simulink library "csc_stm_simplified_temperature_model_collection_lib"  (R2014b)
settings: Solver=ode45  StartTime=0.0  StopTime=10.0  RelTol=1e-3
undefined symbols (not defined in the file or in its folder): stm_celcius_to_bits_slope, stm_tc10_eqn_coefficients, stm_tc11_eqn_coefficients, stm_tc12_eqn_coefficients, stm_tc13_eqn_coefficients, stm_tc14_eqn_coefficients, stm_tc15_eqn_coefficients, stm_tc16_eqn_coefficients, stm_tc17_eqn_coefficients, stm_tc18_eqn_coefficients, stm_tc19_eqn_coefficients, stm_tc1_eqn_coefficients, stm_tc20_eqn_coefficients, stm_tc21_eqn_coefficients, stm_tc22_eqn_coefficients, stm_tc23_eqn_coefficients, stm_tc24_eqn_coefficients, stm_tc25_eqn_coefficients, stm_tc26_eqn_coefficients, stm_tc27_eqn_coefficients, stm_tc28_eqn_coefficients, stm_tc29_eqn_coefficients, stm_tc2_eqn_coefficients, stm_tc30_eqn_coefficients, stm_tc31_eqn_coefficients, stm_tc32_eqn_coefficients, stm_tc33_eqn_coefficients, stm_tc34_eqn_coefficients, stm_tc35_eqn_coefficients, stm_tc36_eqn_coefficients, stm_tc37_eqn_coefficients, stm_tc38_eqn_coefficients, stm_tc39_eqn_coefficients, stm_tc3_eqn_coefficients, stm_tc40_eqn_coefficients, stm_tc41_eqn_coefficients, stm_tc42_eqn_coefficients, stm_tc43_eqn_coefficients, stm_tc44_eqn_coefficients, stm_tc45_eqn_coefficients, stm_tc46_eqn_coefficients, stm_tc47_eqn_coefficients, stm_tc48_eqn_coefficients, stm_tc49_eqn_coefficients, stm_tc4_eqn_coefficients, stm_tc50_eqn_coefficients, stm_tc51_eqn_coefficients, stm_tc52_eqn_coefficients, stm_tc53_eqn_coefficients, stm_tc54_eqn_coefficients, stm_tc55_eqn_coefficients, stm_tc56_eqn_coefficients, stm_tc57_eqn_coefficients, stm_tc58_eqn_coefficients, stm_tc59_eqn_coefficients, stm_tc5_eqn_coefficients, stm_tc60_eqn_coefficients, stm_tc61_eqn_coefficients, stm_tc62_eqn_coefficients, stm_tc63_eqn_coefficients ... (+5)
libraries: csu_stm_simplified_temperature_model_lib x64, util_info_lib x1
settings Model: Creator=escrane  LastModifiedBy=mstewart

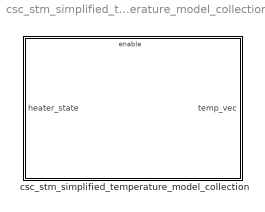
== system csc_stm_simplified_temperature_model_collection_lib ==
  csc_stm_simplified_temperature_model_collection : Subsystem
      mask Display: color('blue');text(0.05, 0.02, 'MoonEx', 'HorizontalAlignment', 'Left', 'VerticalAlignment', 'Bottom');color('red');text(0.95, 0.02, 'Autogenerated', 'HorizontalAlignment', 'Right', 'VerticalAlignment', 'Bottom');

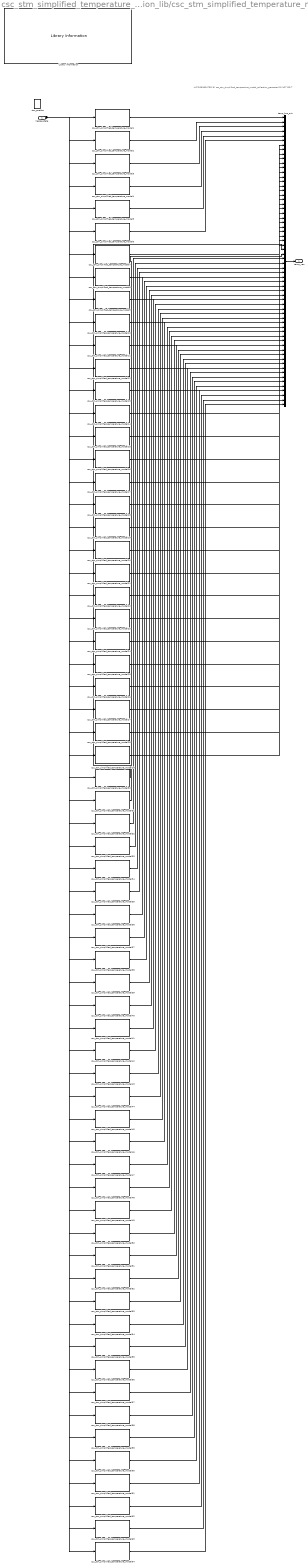
== system csc_stm_simplified_temperature_model_collection_lib/csc_stm_simplified_temperature_model_collection ==
  note: AUTOGENERATED BY csc_stm_simplified_temperature_model_collection_generate
      | DO NOT EDIT
  heater_state : Inport
  stm_enable : EnablePort
  Library Information : util_info_lib/Library Information  owner='NONE'
  csu_stm_simplified_temperature_model1 : csu_stm_simplified_temperature_model_lib/csu_stm_simplified_temperature_model  tc_idx=1  heater_idx=stm_tc1_heater_id  initial_temperature=stm_tc1_initial_temperature  min_temperature=-25  max_temperature=+105  C1=stm_tc1_eqn_coefficients(1)  C2=stm_tc1_eqn_coefficients(2)  C3=stm_tc1_eqn_coefficients(3)  C4=stm_tc1_eqn_coefficients(4)  heater_power=stm_tc1_eqn_coefficients(5)  slope=stm_celcius_to_bits_slope  offset=stm_celcius_to_bits_offset
  csu_stm_simplified_temperature_model10 : csu_stm_simplified_temperature_model_lib/csu_stm_simplified_temperature_model  tc_idx=10  heater_idx=stm_tc10_heater_id  initial_temperature=stm_tc10_initial_temperature  min_temperature=-25  max_temperature=+105  C1=stm_tc10_eqn_coefficients(1)  C2=stm_tc10_eqn_coefficients(2)  C3=stm_tc10_eqn_coefficients(3)  C4=stm_tc10_eqn_coefficients(4)  heater_power=stm_tc10_eqn_coefficients(5)  slope=stm_celcius_to_bits_slope  offset=stm_celcius_to_bits_offset
  csu_stm_simplified_temperature_model11 : csu_stm_simplified_temperature_model_lib/csu_stm_simplified_temperature_model  tc_idx=11  heater_idx=stm_tc11_heater_id  initial_temperature=stm_tc11_initial_temperature  min_temperature=-25  max_temperature=+105  C1=stm_tc11_eqn_coefficients(1)  C2=stm_tc11_eqn_coefficients(2)  C3=stm_tc11_eqn_coefficients(3)  C4=stm_tc11_eqn_coefficients(4)  heater_power=stm_tc11_eqn_coefficients(5)  slope=stm_celcius_to_bits_slope  offset=stm_celcius_to_bits_offset
  csu_stm_simplified_temperature_model12 : csu_stm_simplified_temperature_model_lib/csu_stm_simplified_temperature_model  tc_idx=12  heater_idx=stm_tc12_heater_id  initial_temperature=stm_tc12_initial_temperature  min_temperature=-25  max_temperature=+105  C1=stm_tc12_eqn_coefficients(1)  C2=stm_tc12_eqn_coefficients(2)  C3=stm_tc12_eqn_coefficients(3)  C4=stm_tc12_eqn_coefficients(4)  heater_power=stm_tc12_eqn_coefficients(5)  slope=stm_celcius_to_bits_slope  offset=stm_celcius_to_bits_offset
  csu_stm_simplified_temperature_model13 : csu_stm_simplified_temperature_model_lib/csu_stm_simplified_temperature_model  tc_idx=13  heater_idx=stm_tc13_heater_id  initial_temperature=stm_tc13_initial_temperature  min_temperature=-25  max_temperature=+105  C1=stm_tc13_eqn_coefficients(1)  C2=stm_tc13_eqn_coefficients(2)  C3=stm_tc13_eqn_coefficients(3)  C4=stm_tc13_eqn_coefficients(4)  heater_power=stm_tc13_eqn_coefficients(5)  slope=stm_celcius_to_bits_slope  offset=stm_celcius_to_bits_offset
  csu_stm_simplified_temperature_model14 : csu_stm_simplified_temperature_model_lib/csu_stm_simplified_temperature_model  tc_idx=14  heater_idx=stm_tc14_heater_id  initial_temperature=stm_tc14_initial_temperature  min_temperature=-25  max_temperature=+105  C1=stm_tc14_eqn_coefficients(1)  C2=stm_tc14_eqn_coefficients(2)  C3=stm_tc14_eqn_coefficients(3)  C4=stm_tc14_eqn_coefficients(4)  heater_power=stm_tc14_eqn_coefficients(5)  slope=stm_celcius_to_bits_slope  offset=stm_celcius_to_bits_offset
  csu_stm_simplified_temperature_model15 : csu_stm_simplified_temperature_model_lib/csu_stm_simplified_temperature_model  tc_idx=15  heater_idx=stm_tc15_heater_id  initial_temperature=stm_tc15_initial_temperature  min_temperature=-25  max_temperature=+105  C1=stm_tc15_eqn_coefficients(1)  C2=stm_tc15_eqn_coefficients(2)  C3=stm_tc15_eqn_coefficients(3)  C4=stm_tc15_eqn_coefficients(4)  heater_power=stm_tc15_eqn_coefficients(5)  slope=stm_celcius_to_bits_slope  offset=stm_celcius_to_bits_offset
  csu_stm_simplified_temperature_model16 : csu_stm_simplified_temperature_model_lib/csu_stm_simplified_temperature_model  tc_idx=16  heater_idx=stm_tc16_heater_id  initial_temperature=stm_tc16_initial_temperature  min_temperature=-25  max_temperature=+105  C1=stm_tc16_eqn_coefficients(1)  C2=stm_tc16_eqn_coefficients(2)  C3=stm_tc16_eqn_coefficients(3)  C4=stm_tc16_eqn_coefficients(4)  heater_power=stm_tc16_eqn_coefficients(5)  slope=stm_celcius_to_bits_slope  offset=stm_celcius_to_bits_offset
  csu_stm_simplified_temperature_model17 : csu_stm_simplified_temperature_model_lib/csu_stm_simplified_temperature_model  tc_idx=17  heater_idx=stm_tc17_heater_id  initial_temperature=stm_tc17_initial_temperature  min_temperature=-25  max_temperature=+105  C1=stm_tc17_eqn_coefficients(1)  C2=stm_tc17_eqn_coefficients(2)  C3=stm_tc17_eqn_coefficients(3)  C4=stm_tc17_eqn_coefficients(4)  heater_power=stm_tc17_eqn_coefficients(5)  slope=stm_celcius_to_bits_slope  offset=stm_celcius_to_bits_offset
  csu_stm_simplified_temperature_model18 : csu_stm_simplified_temperature_model_lib/csu_stm_simplified_temperature_model  tc_idx=18  heater_idx=stm_tc18_heater_id  initial_temperature=stm_tc18_initial_temperature  min_temperature=-25  max_temperature=+105  C1=stm_tc18_eqn_coefficients(1)  C2=stm_tc18_eqn_coefficients(2)  C3=stm_tc18_eqn_coefficients(3)  C4=stm_tc18_eqn_coefficients(4)  heater_power=stm_tc18_eqn_coefficients(5)  slope=stm_celcius_to_bits_slope  offset=stm_celcius_to_bits_offset
  csu_stm_simplified_temperature_model19 : csu_stm_simplified_temperature_model_lib/csu_stm_simplified_temperature_model  tc_idx=19  heater_idx=stm_tc19_heater_id  initial_temperature=stm_tc19_initial_temperature  min_temperature=-25  max_temperature=+105  C1=stm_tc19_eqn_coefficients(1)  C2=stm_tc19_eqn_coefficients(2)  C3=stm_tc19_eqn_coefficients(3)  C4=stm_tc19_eqn_coefficients(4)  heater_power=stm_tc19_eqn_coefficients(5)  slope=stm_celcius_to_bits_slope  offset=stm_celcius_to_bits_offset
  csu_stm_simplified_temperature_model2 : csu_stm_simplified_temperature_model_lib/csu_stm_simplified_temperature_model  tc_idx=2  heater_idx=stm_tc2_heater_id  initial_temperature=stm_tc2_initial_temperature  min_temperature=-25  max_temperature=+105  C1=stm_tc2_eqn_coefficients(1)  C2=stm_tc2_eqn_coefficients(2)  C3=stm_tc2_eqn_coefficients(3)  C4=stm_tc2_eqn_coefficients(4)  heater_power=stm_tc2_eqn_coefficients(5)  slope=stm_celcius_to_bits_slope  offset=stm_celcius_to_bits_offset
  csu_stm_simplified_temperature_model20 : csu_stm_simplified_temperature_model_lib/csu_stm_simplified_temperature_model  tc_idx=20  heater_idx=stm_tc20_heater_id  initial_temperature=stm_tc20_initial_temperature  min_temperature=-25  max_temperature=+105  C1=stm_tc20_eqn_coefficients(1)  C2=stm_tc20_eqn_coefficients(2)  C3=stm_tc20_eqn_coefficients(3)  C4=stm_tc20_eqn_coefficients(4)  heater_power=stm_tc20_eqn_coefficients(5)  slope=stm_celcius_to_bits_slope  offset=stm_celcius_to_bits_offset
  csu_stm_simplified_temperature_model21 : csu_stm_simplified_temperature_model_lib/csu_stm_simplified_temperature_model  tc_idx=21  heater_idx=stm_tc21_heater_id  initial_temperature=stm_tc21_initial_temperature  min_temperature=-25  max_temperature=+105  C1=stm_tc21_eqn_coefficients(1)  C2=stm_tc21_eqn_coefficients(2)  C3=stm_tc21_eqn_coefficients(3)  C4=stm_tc21_eqn_coefficients(4)  heater_power=stm_tc21_eqn_coefficients(5)  slope=stm_celcius_to_bits_slope  offset=stm_celcius_to_bits_offset
  csu_stm_simplified_temperature_model22 : csu_stm_simplified_temperature_model_lib/csu_stm_simplified_temperature_model  tc_idx=22  heater_idx=stm_tc22_heater_id  initial_temperature=stm_tc22_initial_temperature  min_temperature=-25  max_temperature=+105  C1=stm_tc22_eqn_coefficients(1)  C2=stm_tc22_eqn_coefficients(2)  C3=stm_tc22_eqn_coefficients(3)  C4=stm_tc22_eqn_coefficients(4)  heater_power=stm_tc22_eqn_coefficients(5)  slope=stm_celcius_to_bits_slope  offset=stm_celcius_to_bits_offset
  csu_stm_simplified_temperature_model23 : csu_stm_simplified_temperature_model_lib/csu_stm_simplified_temperature_model  tc_idx=23  heater_idx=stm_tc23_heater_id  initial_temperature=stm_tc23_initial_temperature  min_temperature=-25  max_temperature=+105  C1=stm_tc23_eqn_coefficients(1)  C2=stm_tc23_eqn_coefficients(2)  C3=stm_tc23_eqn_coefficients(3)  C4=stm_tc23_eqn_coefficients(4)  heater_power=stm_tc23_eqn_coefficients(5)  slope=stm_celcius_to_bits_slope  offset=stm_celcius_to_bits_offset
  csu_stm_simplified_temperature_model24 : csu_stm_simplified_temperature_model_lib/csu_stm_simplified_temperature_model  tc_idx=24  heater_idx=stm_tc24_heater_id  initial_temperature=stm_tc24_initial_temperature  min_temperature=-25  max_temperature=+105  C1=stm_tc24_eqn_coefficients(1)  C2=stm_tc24_eqn_coefficients(2)  C3=stm_tc24_eqn_coefficients(3)  C4=stm_tc24_eqn_coefficients(4)  heater_power=stm_tc24_eqn_coefficients(5)  slope=stm_celcius_to_bits_slope  offset=stm_celcius_to_bits_offset
  csu_stm_simplified_temperature_model25 : csu_stm_simplified_temperature_model_lib/csu_stm_simplified_temperature_model  tc_idx=25  heater_idx=stm_tc25_heater_id  initial_temperature=stm_tc25_initial_temperature  min_temperature=-25  max_temperature=+105  C1=stm_tc25_eqn_coefficients(1)  C2=stm_tc25_eqn_coefficients(2)  C3=stm_tc25_eqn_coefficients(3)  C4=stm_tc25_eqn_coefficients(4)  heater_power=stm_tc25_eqn_coefficients(5)  slope=stm_celcius_to_bits_slope  offset=stm_celcius_to_bits_offset
  csu_stm_simplified_temperature_model26 : csu_stm_simplified_temperature_model_lib/csu_stm_simplified_temperature_model  tc_idx=26  heater_idx=stm_tc26_heater_id  initial_temperature=stm_tc26_initial_temperature  min_temperature=-25  max_temperature=+105  C1=stm_tc26_eqn_coefficients(1)  C2=stm_tc26_eqn_coefficients(2)  C3=stm_tc26_eqn_coefficients(3)  C4=stm_tc26_eqn_coefficients(4)  heater_power=stm_tc26_eqn_coefficients(5)  slope=stm_celcius_to_bits_slope  offset=stm_celcius_to_bits_offset
  csu_stm_simplified_temperature_model27 : csu_stm_simplified_temperature_model_lib/csu_stm_simplified_temperature_model  tc_idx=27  heater_idx=stm_tc27_heater_id  initial_temperature=stm_tc27_initial_temperature  min_temperature=-25  max_temperature=+105  C1=stm_tc27_eqn_coefficients(1)  C2=stm_tc27_eqn_coefficients(2)  C3=stm_tc27_eqn_coefficients(3)  C4=stm_tc27_eqn_coefficients(4)  heater_power=stm_tc27_eqn_coefficients(5)  slope=stm_celcius_to_bits_slope  offset=stm_celcius_to_bits_offset
  csu_stm_simplified_temperature_model28 : csu_stm_simplified_temperature_model_lib/csu_stm_simplified_temperature_model  tc_idx=28  heater_idx=stm_tc28_heater_id  initial_temperature=stm_tc28_initial_temperature  min_temperature=-25  max_temperature=+105  C1=stm_tc28_eqn_coefficients(1)  C2=stm_tc28_eqn_coefficients(2)  C3=stm_tc28_eqn_coefficients(3)  C4=stm_tc28_eqn_coefficients(4)  heater_power=stm_tc28_eqn_coefficients(5)  slope=stm_celcius_to_bits_slope  offset=stm_celcius_to_bits_offset
  csu_stm_simplified_temperature_model29 : csu_stm_simplified_temperature_model_lib/csu_stm_simplified_temperature_model  tc_idx=29  heater_idx=stm_tc29_heater_id  initial_temperature=stm_tc29_initial_temperature  min_temperature=-25  max_temperature=+105  C1=stm_tc29_eqn_coefficients(1)  C2=stm_tc29_eqn_coefficients(2)  C3=stm_tc29_eqn_coefficients(3)  C4=stm_tc29_eqn_coefficients(4)  heater_power=stm_tc29_eqn_coefficients(5)  slope=stm_celcius_to_bits_slope  offset=stm_celcius_to_bits_offset
  csu_stm_simplified_temperature_model3 : csu_stm_simplified_temperature_model_lib/csu_stm_simplified_temperature_model  tc_idx=3  heater_idx=stm_tc3_heater_id  initial_temperature=stm_tc3_initial_temperature  min_temperature=-25  max_temperature=+105  C1=stm_tc3_eqn_coefficients(1)  C2=stm_tc3_eqn_coefficients(2)  C3=stm_tc3_eqn_coefficients(3)  C4=stm_tc3_eqn_coefficients(4)  heater_power=stm_tc3_eqn_coefficients(5)  slope=stm_celcius_to_bits_slope  offset=stm_celcius_to_bits_offset
  csu_stm_simplified_temperature_model30 : csu_stm_simplified_temperature_model_lib/csu_stm_simplified_temperature_model  tc_idx=30  heater_idx=stm_tc30_heater_id  initial_temperature=stm_tc30_initial_temperature  min_temperature=-25  max_temperature=+105  C1=stm_tc30_eqn_coefficients(1)  C2=stm_tc30_eqn_coefficients(2)  C3=stm_tc30_eqn_coefficients(3)  C4=stm_tc30_eqn_coefficients(4)  heater_power=stm_tc30_eqn_coefficients(5)  slope=stm_celcius_to_bits_slope  offset=stm_celcius_to_bits_offset
  csu_stm_simplified_temperature_model31 : csu_stm_simplified_temperature_model_lib/csu_stm_simplified_temperature_model  tc_idx=31  heater_idx=stm_tc31_heater_id  initial_temperature=stm_tc31_initial_temperature  min_temperature=-25  max_temperature=+105  C1=stm_tc31_eqn_coefficients(1)  C2=stm_tc31_eqn_coefficients(2)  C3=stm_tc31_eqn_coefficients(3)  C4=stm_tc31_eqn_coefficients(4)  heater_power=stm_tc31_eqn_coefficients(5)  slope=stm_celcius_to_bits_slope  offset=stm_celcius_to_bits_offset
  csu_stm_simplified_temperature_model32 : csu_stm_simplified_temperature_model_lib/csu_stm_simplified_temperature_model  tc_idx=32  heater_idx=stm_tc32_heater_id  initial_temperature=stm_tc32_initial_temperature  min_temperature=-25  max_temperature=+105  C1=stm_tc32_eqn_coefficients(1)  C2=stm_tc32_eqn_coefficients(2)  C3=stm_tc32_eqn_coefficients(3)  C4=stm_tc32_eqn_coefficients(4)  heater_power=stm_tc32_eqn_coefficients(5)  slope=stm_celcius_to_bits_slope  offset=stm_celcius_to_bits_offset
  csu_stm_simplified_temperature_model33 : csu_stm_simplified_temperature_model_lib/csu_stm_simplified_temperature_model  tc_idx=33  heater_idx=stm_tc33_heater_id  initial_temperature=stm_tc33_initial_temperature  min_temperature=-25  max_temperature=+105  C1=stm_tc33_eqn_coefficients(1)  C2=stm_tc33_eqn_coefficients(2)  C3=stm_tc33_eqn_coefficients(3)  C4=stm_tc33_eqn_coefficients(4)  heater_power=stm_tc33_eqn_coefficients(5)  slope=stm_celcius_to_bits_slope  offset=stm_celcius_to_bits_offset
  csu_stm_simplified_temperature_model34 : csu_stm_simplified_temperature_model_lib/csu_stm_simplified_temperature_model  tc_idx=34  heater_idx=stm_tc34_heater_id  initial_temperature=stm_tc34_initial_temperature  min_temperature=-25  max_temperature=+105  C1=stm_tc34_eqn_coefficients(1)  C2=stm_tc34_eqn_coefficients(2)  C3=stm_tc34_eqn_coefficients(3)  C4=stm_tc34_eqn_coefficients(4)  heater_power=stm_tc34_eqn_coefficients(5)  slope=stm_celcius_to_bits_slope  offset=stm_celcius_to_bits_offset
  csu_stm_simplified_temperature_model35 : csu_stm_simplified_temperature_model_lib/csu_stm_simplified_temperature_model  tc_idx=35  heater_idx=stm_tc35_heater_id  initial_temperature=stm_tc35_initial_temperature  min_temperature=-25  max_temperature=+105  C1=stm_tc35_eqn_coefficients(1)  C2=stm_tc35_eqn_coefficients(2)  C3=stm_tc35_eqn_coefficients(3)  C4=stm_tc35_eqn_coefficients(4)  heater_power=stm_tc35_eqn_coefficients(5)  slope=stm_celcius_to_bits_slope  offset=stm_celcius_to_bits_offset
  csu_stm_simplified_temperature_model36 : csu_stm_simplified_temperature_model_lib/csu_stm_simplified_temperature_model  tc_idx=36  heater_idx=stm_tc36_heater_id  initial_temperature=stm_tc36_initial_temperature  min_temperature=-25  max_temperature=+105  C1=stm_tc36_eqn_coefficients(1)  C2=stm_tc36_eqn_coefficients(2)  C3=stm_tc36_eqn_coefficients(3)  C4=stm_tc36_eqn_coefficients(4)  heater_power=stm_tc36_eqn_coefficients(5)  slope=stm_celcius_to_bits_slope  offset=stm_celcius_to_bits_offset
  csu_stm_simplified_temperature_model37 : csu_stm_simplified_temperature_model_lib/csu_stm_simplified_temperature_model  tc_idx=37  heater_idx=stm_tc37_heater_id  initial_temperature=stm_tc37_initial_temperature  min_temperature=-25  max_temperature=+105  C1=stm_tc37_eqn_coefficients(1)  C2=stm_tc37_eqn_coefficients(2)  C3=stm_tc37_eqn_coefficients(3)  C4=stm_tc37_eqn_coefficients(4)  heater_power=stm_tc37_eqn_coefficients(5)  slope=stm_celcius_to_bits_slope  offset=stm_celcius_to_bits_offset
  csu_stm_simplified_temperature_model38 : csu_stm_simplified_temperature_model_lib/csu_stm_simplified_temperature_model  tc_idx=38  heater_idx=stm_tc38_heater_id  initial_temperature=stm_tc38_initial_temperature  min_temperature=-25  max_temperature=+105  C1=stm_tc38_eqn_coefficients(1)  C2=stm_tc38_eqn_coefficients(2)  C3=stm_tc38_eqn_coefficients(3)  C4=stm_tc38_eqn_coefficients(4)  heater_power=stm_tc38_eqn_coefficients(5)  slope=stm_celcius_to_bits_slope  offset=stm_celcius_to_bits_offset
  csu_stm_simplified_temperature_model39 : csu_stm_simplified_temperature_model_lib/csu_stm_simplified_temperature_model  tc_idx=39  heater_idx=stm_tc39_heater_id  initial_temperature=stm_tc39_initial_temperature  min_temperature=-25  max_temperature=+105  C1=stm_tc39_eqn_coefficients(1)  C2=stm_tc39_eqn_coefficients(2)  C3=stm_tc39_eqn_coefficients(3)  C4=stm_tc39_eqn_coefficients(4)  heater_power=stm_tc39_eqn_coefficients(5)  slope=stm_celcius_to_bits_slope  offset=stm_celcius_to_bits_offset
  csu_stm_simplified_temperature_model4 : csu_stm_simplified_temperature_model_lib/csu_stm_simplified_temperature_model  tc_idx=4  heater_idx=stm_tc4_heater_id  initial_temperature=stm_tc4_initial_temperature  min_temperature=-25  max_temperature=+105  C1=stm_tc4_eqn_coefficients(1)  C2=stm_tc4_eqn_coefficients(2)  C3=stm_tc4_eqn_coefficients(3)  C4=stm_tc4_eqn_coefficients(4)  heater_power=stm_tc4_eqn_coefficients(5)  slope=stm_celcius_to_bits_slope  offset=stm_celcius_to_bits_offset
  csu_stm_simplified_temperature_model40 : csu_stm_simplified_temperature_model_lib/csu_stm_simplified_temperature_model  tc_idx=40  heater_idx=stm_tc40_heater_id  initial_temperature=stm_tc40_initial_temperature  min_temperature=-25  max_temperature=+105  C1=stm_tc40_eqn_coefficients(1)  C2=stm_tc40_eqn_coefficients(2)  C3=stm_tc40_eqn_coefficients(3)  C4=stm_tc40_eqn_coefficients(4)  heater_power=stm_tc40_eqn_coefficients(5)  slope=stm_celcius_to_bits_slope  offset=stm_celcius_to_bits_offset
  csu_stm_simplified_temperature_model41 : csu_stm_simplified_temperature_model_lib/csu_stm_simplified_temperature_model  tc_idx=41  heater_idx=stm_tc41_heater_id  initial_temperature=stm_tc41_initial_temperature  min_temperature=-25  max_temperature=+105  C1=stm_tc41_eqn_coefficients(1)  C2=stm_tc41_eqn_coefficients(2)  C3=stm_tc41_eqn_coefficients(3)  C4=stm_tc41_eqn_coefficients(4)  heater_power=stm_tc41_eqn_coefficients(5)  slope=stm_celcius_to_bits_slope  offset=stm_celcius_to_bits_offset
  csu_stm_simplified_temperature_model42 : csu_stm_simplified_temperature_model_lib/csu_stm_simplified_temperature_model  tc_idx=42  heater_idx=stm_tc42_heater_id  initial_temperature=stm_tc42_initial_temperature  min_temperature=-25  max_temperature=+105  C1=stm_tc42_eqn_coefficients(1)  C2=stm_tc42_eqn_coefficients(2)  C3=stm_tc42_eqn_coefficients(3)  C4=stm_tc42_eqn_coefficients(4)  heater_power=stm_tc42_eqn_coefficients(5)  slope=stm_celcius_to_bits_slope  offset=stm_celcius_to_bits_offset
  csu_stm_simplified_temperature_model43 : csu_stm_simplified_temperature_model_lib/csu_stm_simplified_temperature_model  tc_idx=43  heater_idx=stm_tc43_heater_id  initial_temperature=stm_tc43_initial_temperature  min_temperature=-25  max_temperature=+105  C1=stm_tc43_eqn_coefficients(1)  C2=stm_tc43_eqn_coefficients(2)  C3=stm_tc43_eqn_coefficients(3)  C4=stm_tc43_eqn_coefficients(4)  heater_power=stm_tc43_eqn_coefficients(5)  slope=stm_celcius_to_bits_slope  offset=stm_celcius_to_bits_offset
  csu_stm_simplified_temperature_model44 : csu_stm_simplified_temperature_model_lib/csu_stm_simplified_temperature_model  tc_idx=44  heater_idx=stm_tc44_heater_id  initial_temperature=stm_tc44_initial_temperature  min_temperature=-25  max_temperature=+105  C1=stm_tc44_eqn_coefficients(1)  C2=stm_tc44_eqn_coefficients(2)  C3=stm_tc44_eqn_coefficients(3)  C4=stm_tc44_eqn_coefficients(4)  heater_power=stm_tc44_eqn_coefficients(5)  slope=stm_celcius_to_bits_slope  offset=stm_celcius_to_bits_offset
  csu_stm_simplified_temperature_model45 : csu_stm_simplified_temperature_model_lib/csu_stm_simplified_temperature_model  tc_idx=45  heater_idx=stm_tc45_heater_id  initial_temperature=stm_tc45_initial_temperature  min_temperature=-25  max_temperature=+105  C1=stm_tc45_eqn_coefficients(1)  C2=stm_tc45_eqn_coefficients(2)  C3=stm_tc45_eqn_coefficients(3)  C4=stm_tc45_eqn_coefficients(4)  heater_power=stm_tc45_eqn_coefficients(5)  slope=stm_celcius_to_bits_slope  offset=stm_celcius_to_bits_offset
  csu_stm_simplified_temperature_model46 : csu_stm_simplified_temperature_model_lib/csu_stm_simplified_temperature_model  tc_idx=46  heater_idx=stm_tc46_heater_id  initial_temperature=stm_tc46_initial_temperature  min_temperature=-25  max_temperature=+105  C1=stm_tc46_eqn_coefficients(1)  C2=stm_tc46_eqn_coefficients(2)  C3=stm_tc46_eqn_coefficients(3)  C4=stm_tc46_eqn_coefficients(4)  heater_power=stm_tc46_eqn_coefficients(5)  slope=stm_celcius_to_bits_slope  offset=stm_celcius_to_bits_offset
  csu_stm_simplified_temperature_model47 : csu_stm_simplified_temperature_model_lib/csu_stm_simplified_temperature_model  tc_idx=47  heater_idx=stm_tc47_heater_id  initial_temperature=stm_tc47_initial_temperature  min_temperature=-25  max_temperature=+105  C1=stm_tc47_eqn_coefficients(1)  C2=stm_tc47_eqn_coefficients(2)  C3=stm_tc47_eqn_coefficients(3)  C4=stm_tc47_eqn_coefficients(4)  heater_power=stm_tc47_eqn_coefficients(5)  slope=stm_celcius_to_bits_slope  offset=stm_celcius_to_bits_offset
  csu_stm_simplified_temperature_model48 : csu_stm_simplified_temperature_model_lib/csu_stm_simplified_temperature_model  tc_idx=48  heater_idx=stm_tc48_heater_id  initial_temperature=stm_tc48_initial_temperature  min_temperature=-25  max_temperature=+105  C1=stm_tc48_eqn_coefficients(1)  C2=stm_tc48_eqn_coefficients(2)  C3=stm_tc48_eqn_coefficients(3)  C4=stm_tc48_eqn_coefficients(4)  heater_power=stm_tc48_eqn_coefficients(5)  slope=stm_celcius_to_bits_slope  offset=stm_celcius_to_bits_offset
  csu_stm_simplified_temperature_model49 : csu_stm_simplified_temperature_model_lib/csu_stm_simplified_temperature_model  tc_idx=49  heater_idx=stm_tc49_heater_id  initial_temperature=stm_tc49_initial_temperature  min_temperature=-25  max_temperature=+105  C1=stm_tc49_eqn_coefficients(1)  C2=stm_tc49_eqn_coefficients(2)  C3=stm_tc49_eqn_coefficients(3)  C4=stm_tc49_eqn_coefficients(4)  heater_power=stm_tc49_eqn_coefficients(5)  slope=stm_celcius_to_bits_slope  offset=stm_celcius_to_bits_offset
  csu_stm_simplified_temperature_model5 : csu_stm_simplified_temperature_model_lib/csu_stm_simplified_temperature_model  tc_idx=5  heater_idx=stm_tc5_heater_id  initial_temperature=stm_tc5_initial_temperature  min_temperature=-25  max_temperature=+105  C1=stm_tc5_eqn_coefficients(1)  C2=stm_tc5_eqn_coefficients(2)  C3=stm_tc5_eqn_coefficients(3)  C4=stm_tc5_eqn_coefficients(4)  heater_power=stm_tc5_eqn_coefficients(5)  slope=stm_celcius_to_bits_slope  offset=stm_celcius_to_bits_offset
  csu_stm_simplified_temperature_model50 : csu_stm_simplified_temperature_model_lib/csu_stm_simplified_temperature_model  tc_idx=50  heater_idx=stm_tc50_heater_id  initial_temperature=stm_tc50_initial_temperature  min_temperature=-25  max_temperature=+105  C1=stm_tc50_eqn_coefficients(1)  C2=stm_tc50_eqn_coefficients(2)  C3=stm_tc50_eqn_coefficients(3)  C4=stm_tc50_eqn_coefficients(4)  heater_power=stm_tc50_eqn_coefficients(5)  slope=stm_celcius_to_bits_slope  offset=stm_celcius_to_bits_offset
  csu_stm_simplified_temperature_model51 : csu_stm_simplified_temperature_model_lib/csu_stm_simplified_temperature_model  tc_idx=51  heater_idx=stm_tc51_heater_id  initial_temperature=stm_tc51_initial_temperature  min_temperature=-25  max_temperature=+105  C1=stm_tc51_eqn_coefficients(1)  C2=stm_tc51_eqn_coefficients(2)  C3=stm_tc51_eqn_coefficients(3)  C4=stm_tc51_eqn_coefficients(4)  heater_power=stm_tc51_eqn_coefficients(5)  slope=stm_celcius_to_bits_slope  offset=stm_celcius_to_bits_offset
  csu_stm_simplified_temperature_model52 : csu_stm_simplified_temperature_model_lib/csu_stm_simplified_temperature_model  tc_idx=52  heater_idx=stm_tc52_heater_id  initial_temperature=stm_tc52_initial_temperature  min_temperature=-25  max_temperature=+105  C1=stm_tc52_eqn_coefficients(1)  C2=stm_tc52_eqn_coefficients(2)  C3=stm_tc52_eqn_coefficients(3)  C4=stm_tc52_eqn_coefficients(4)  heater_power=stm_tc52_eqn_coefficients(5)  slope=stm_celcius_to_bits_slope  offset=stm_celcius_to_bits_offset
  csu_stm_simplified_temperature_model53 : csu_stm_simplified_temperature_model_lib/csu_stm_simplified_temperature_model  tc_idx=53  heater_idx=stm_tc53_heater_id  initial_temperature=stm_tc53_initial_temperature  min_temperature=-25  max_temperature=+105  C1=stm_tc53_eqn_coefficients(1)  C2=stm_tc53_eqn_coefficients(2)  C3=stm_tc53_eqn_coefficients(3)  C4=stm_tc53_eqn_coefficients(4)  heater_power=stm_tc53_eqn_coefficients(5)  slope=stm_celcius_to_bits_slope  offset=stm_celcius_to_bits_offset
  csu_stm_simplified_temperature_model54 : csu_stm_simplified_temperature_model_lib/csu_stm_simplified_temperature_model  tc_idx=54  heater_idx=stm_tc54_heater_id  initial_temperature=stm_tc54_initial_temperature  min_temperature=-25  max_temperature=+105  C1=stm_tc54_eqn_coefficients(1)  C2=stm_tc54_eqn_coefficients(2)  C3=stm_tc54_eqn_coefficients(3)  C4=stm_tc54_eqn_coefficients(4)  heater_power=stm_tc54_eqn_coefficients(5)  slope=stm_celcius_to_bits_slope  offset=stm_celcius_to_bits_offset
  csu_stm_simplified_temperature_model55 : csu_stm_simplified_temperature_model_lib/csu_stm_simplified_temperature_model  tc_idx=55  heater_idx=stm_tc55_heater_id  initial_temperature=stm_tc55_initial_temperature  min_temperature=-25  max_temperature=+105  C1=stm_tc55_eqn_coefficients(1)  C2=stm_tc55_eqn_coefficients(2)  C3=stm_tc55_eqn_coefficients(3)  C4=stm_tc55_eqn_coefficients(4)  heater_power=stm_tc55_eqn_coefficients(5)  slope=stm_celcius_to_bits_slope  offset=stm_celcius_to_bits_offset
  csu_stm_simplified_temperature_model56 : csu_stm_simplified_temperature_model_lib/csu_stm_simplified_temperature_model  tc_idx=56  heater_idx=stm_tc56_heater_id  initial_temperature=stm_tc56_initial_temperature  min_temperature=-25  max_temperature=+105  C1=stm_tc56_eqn_coefficients(1)  C2=stm_tc56_eqn_coefficients(2)  C3=stm_tc56_eqn_coefficients(3)  C4=stm_tc56_eqn_coefficients(4)  heater_power=stm_tc56_eqn_coefficients(5)  slope=stm_celcius_to_bits_slope  offset=stm_celcius_to_bits_offset
  csu_stm_simplified_temperature_model57 : csu_stm_simplified_temperature_model_lib/csu_stm_simplified_temperature_model  tc_idx=57  heater_idx=stm_tc57_heater_id  initial_temperature=stm_tc57_initial_temperature  min_temperature=-25  max_temperature=+105  C1=stm_tc57_eqn_coefficients(1)  C2=stm_tc57_eqn_coefficients(2)  C3=stm_tc57_eqn_coefficients(3)  C4=stm_tc57_eqn_coefficients(4)  heater_power=stm_tc57_eqn_coefficients(5)  slope=stm_celcius_to_bits_slope  offset=stm_celcius_to_bits_offset
  csu_stm_simplified_temperature_model58 : csu_stm_simplified_temperature_model_lib/csu_stm_simplified_temperature_model  tc_idx=58  heater_idx=stm_tc58_heater_id  initial_temperature=stm_tc58_initial_temperature  min_temperature=-25  max_temperature=+105  C1=stm_tc58_eqn_coefficients(1)  C2=stm_tc58_eqn_coefficients(2)  C3=stm_tc58_eqn_coefficients(3)  C4=stm_tc58_eqn_coefficients(4)  heater_power=stm_tc58_eqn_coefficients(5)  slope=stm_celcius_to_bits_slope  offset=stm_celcius_to_bits_offset
  csu_stm_simplified_temperature_model59 : csu_stm_simplified_temperature_model_lib/csu_stm_simplified_temperature_model  tc_idx=59  heater_idx=stm_tc59_heater_id  initial_temperature=stm_tc59_initial_temperature  min_temperature=-25  max_temperature=+105  C1=stm_tc59_eqn_coefficients(1)  C2=stm_tc59_eqn_coefficients(2)  C3=stm_tc59_eqn_coefficients(3)  C4=stm_tc59_eqn_coefficients(4)  heater_power=stm_tc59_eqn_coefficients(5)  slope=stm_celcius_to_bits_slope  offset=stm_celcius_to_bits_offset
  csu_stm_simplified_temperature_model6 : csu_stm_simplified_temperature_model_lib/csu_stm_simplified_temperature_model  tc_idx=6  heater_idx=stm_tc6_heater_id  initial_temperature=stm_tc6_initial_temperature  min_temperature=-25  max_temperature=+105  C1=stm_tc6_eqn_coefficients(1)  C2=stm_tc6_eqn_coefficients(2)  C3=stm_tc6_eqn_coefficients(3)  C4=stm_tc6_eqn_coefficients(4)  heater_power=stm_tc6_eqn_coefficients(5)  slope=stm_celcius_to_bits_slope  offset=stm_celcius_to_bits_offset
  csu_stm_simplified_temperature_model60 : csu_stm_simplified_temperature_model_lib/csu_stm_simplified_temperature_model  tc_idx=60  heater_idx=stm_tc60_heater_id  initial_temperature=stm_tc60_initial_temperature  min_temperature=-25  max_temperature=+105  C1=stm_tc60_eqn_coefficients(1)  C2=stm_tc60_eqn_coefficients(2)  C3=stm_tc60_eqn_coefficients(3)  C4=stm_tc60_eqn_coefficients(4)  heater_power=stm_tc60_eqn_coefficients(5)  slope=stm_celcius_to_bits_slope  offset=stm_celcius_to_bits_offset
  csu_stm_simplified_temperature_model61 : csu_stm_simplified_temperature_model_lib/csu_stm_simplified_temperature_model  tc_idx=61  heater_idx=stm_tc61_heater_id  initial_temperature=stm_tc61_initial_temperature  min_temperature=-25  max_temperature=+105  C1=stm_tc61_eqn_coefficients(1)  C2=stm_tc61_eqn_coefficients(2)  C3=stm_tc61_eqn_coefficients(3)  C4=stm_tc61_eqn_coefficients(4)  heater_power=stm_tc61_eqn_coefficients(5)  slope=stm_celcius_to_bits_slope  offset=stm_celcius_to_bits_offset
  csu_stm_simplified_temperature_model62 : csu_stm_simplified_temperature_model_lib/csu_stm_simplified_temperature_model  tc_idx=62  heater_idx=stm_tc62_heater_id  initial_temperature=stm_tc62_initial_temperature  min_temperature=-25  max_temperature=+105  C1=stm_tc62_eqn_coefficients(1)  C2=stm_tc62_eqn_coefficients(2)  C3=stm_tc62_eqn_coefficients(3)  C4=stm_tc62_eqn_coefficients(4)  heater_power=stm_tc62_eqn_coefficients(5)  slope=stm_celcius_to_bits_slope  offset=stm_celcius_to_bits_offset
  csu_stm_simplified_temperature_model63 : csu_stm_simplified_temperature_model_lib/csu_stm_simplified_temperature_model  tc_idx=63  heater_idx=stm_tc63_heater_id  initial_temperature=stm_tc63_initial_temperature  min_temperature=-25  max_temperature=+105  C1=stm_tc63_eqn_coefficients(1)  C2=stm_tc63_eqn_coefficients(2)  C3=stm_tc63_eqn_coefficients(3)  C4=stm_tc63_eqn_coefficients(4)  heater_power=stm_tc63_eqn_coefficients(5)  slope=stm_celcius_to_bits_slope  offset=stm_celcius_to_bits_offset
  csu_stm_simplified_temperature_model64 : csu_stm_simplified_temperature_model_lib/csu_stm_simplified_temperature_model  tc_idx=64  heater_idx=stm_tc64_heater_id  initial_temperature=stm_tc64_initial_temperature  min_temperature=-25  max_temperature=+105  C1=stm_tc64_eqn_coefficients(1)  C2=stm_tc64_eqn_coefficients(2)  C3=stm_tc64_eqn_coefficients(3)  C4=stm_tc64_eqn_coefficients(4)  heater_power=stm_tc64_eqn_coefficients(5)  slope=stm_celcius_to_bits_slope  offset=stm_celcius_to_bits_offset
  csu_stm_simplified_temperature_model7 : csu_stm_simplified_temperature_model_lib/csu_stm_simplified_temperature_model  tc_idx=7  heater_idx=stm_tc7_heater_id  initial_temperature=stm_tc7_initial_temperature  min_temperature=-25  max_temperature=+105  C1=stm_tc7_eqn_coefficients(1)  C2=stm_tc7_eqn_coefficients(2)  C3=stm_tc7_eqn_coefficients(3)  C4=stm_tc7_eqn_coefficients(4)  heater_power=stm_tc7_eqn_coefficients(5)  slope=stm_celcius_to_bits_slope  offset=stm_celcius_to_bits_offset
  csu_stm_simplified_temperature_model8 : csu_stm_simplified_temperature_model_lib/csu_stm_simplified_temperature_model  tc_idx=8  heater_idx=stm_tc8_heater_id  initial_temperature=stm_tc8_initial_temperature  min_temperature=-25  max_temperature=+105  C1=stm_tc8_eqn_coefficients(1)  C2=stm_tc8_eqn_coefficients(2)  C3=stm_tc8_eqn_coefficients(3)  C4=stm_tc8_eqn_coefficients(4)  heater_power=stm_tc8_eqn_coefficients(5)  slope=stm_celcius_to_bits_slope  offset=stm_celcius_to_bits_offset
  csu_stm_simplified_temperature_model9 : csu_stm_simplified_temperature_model_lib/csu_stm_simplified_temperature_model  tc_idx=9  heater_idx=stm_tc9_heater_id  initial_temperature=stm_tc9_initial_temperature  min_temperature=-25  max_temperature=+105  C1=stm_tc9_eqn_coefficients(1)  C2=stm_tc9_eqn_coefficients(2)  C3=stm_tc9_eqn_coefficients(3)  C4=stm_tc9_eqn_coefficients(4)  heater_power=stm_tc9_eqn_coefficients(5)  slope=stm_celcius_to_bits_slope  offset=stm_celcius_to_bits_offset
  temp_bus_out : BusCreator  Inputs=64
  temp_vec : Outport
  wires:
  temp_bus_out/1 -> temp_vec/1
  heater_state/1 -> csu_stm_simplified_temperature_model64/1, csu_stm_simplified_temperature_model63/1, csu_stm_simplified_temperature_model62/1, csu_stm_simplified_temperature_model61/1, csu_stm_simplified_temperature_model60/1, csu_stm_simplified_temperature_model59/1, csu_stm_simplified_temperature_model58/1, csu_stm_simplified_temperature_model57/1, csu_stm_simplified_temperature_model56/1, csu_stm_simplified_temperature_model55/1, csu_stm_simplified_temperature_model54/1, csu_stm_simplified_temperature_model53/1, csu_stm_simplified_temperature_model52/1, csu_stm_simplified_temperature_model51/1, csu_stm_simplified_temperature_model50/1, csu_stm_simplified_temperature_model49/1, csu_stm_simplified_temperature_model48/1, csu_stm_simplified_temperature_model47/1, csu_stm_simplified_temperature_model46/1, csu_stm_simplified_temperature_model45/1, csu_stm_simplified_temperature_model44/1, csu_stm_simplified_temperature_model43/1, csu_stm_simplified_temperature_model42/1, csu_stm_simplified_temperature_model41/1, csu_stm_simplified_temperature_model40/1, csu_stm_simplified_temperature_model39/1, csu_stm_simplified_temperature_model38/1, csu_stm_simplified_temperature_model37/1, csu_stm_simplified_temperature_model36/1, csu_stm_simplified_temperature_model35/1, csu_stm_simplified_temperature_model34/1, csu_stm_simplified_temperature_model33/1, csu_stm_simplified_temperature_model32/1, csu_stm_simplified_temperature_model31/1, csu_stm_simplified_temperature_model30/1, csu_stm_simplified_temperature_model29/1, csu_stm_simplified_temperature_model28/1, csu_stm_simplified_temperature_model27/1, csu_stm_simplified_temperature_model26/1, csu_stm_simplified_temperature_model25/1, csu_stm_simplified_temperature_model24/1, csu_stm_simplified_temperature_model23/1, csu_stm_simplified_temperature_model22/1, csu_stm_simplified_temperature_model21/1, csu_stm_simplified_temperature_model20/1, csu_stm_simplified_temperature_model19/1, csu_stm_simplified_temperature_model18/1, csu_stm_simplified_temperature_model17/1, csu_stm_simplified_temperature_model16/1, csu_stm_simplified_temperature_model15/1, csu_stm_simplified_temperature_model14/1, csu_stm_simplified_temperature_model13/1, csu_stm_simplified_temperature_model12/1, csu_stm_simplified_temperature_model11/1, csu_stm_simplified_temperature_model10/1, csu_stm_simplified_temperature_model9/1, csu_stm_simplified_temperature_model8/1, csu_stm_simplified_temperature_model7/1, csu_stm_simplified_temperature_model6/1, csu_stm_simplified_temperature_model5/1, csu_stm_simplified_temperature_model4/1, csu_stm_simplified_temperature_model3/1, csu_stm_simplified_temperature_model2/1, csu_stm_simplified_temperature_model1/1
  csu_stm_simplified_temperature_model64/1 -> temp_bus_out/64  "temp_sense_64"
  csu_stm_simplified_temperature_model63/1 -> temp_bus_out/63  "temp_sense_63"
  csu_stm_simplified_temperature_model62/1 -> temp_bus_out/62  "temp_sense_62"
  csu_stm_simplified_temperature_model61/1 -> temp_bus_out/61  "temp_sense_61"
  csu_stm_simplified_temperature_model60/1 -> temp_bus_out/60  "temp_sense_60"
  csu_stm_simplified_temperature_model59/1 -> temp_bus_out/59  "temp_sense_59"
  csu_stm_simplified_temperature_model58/1 -> temp_bus_out/58  "temp_sense_58"
  csu_stm_simplified_temperature_model57/1 -> temp_bus_out/57  "temp_sense_57"
  csu_stm_simplified_temperature_model56/1 -> temp_bus_out/56  "temp_sense_56"
  csu_stm_simplified_temperature_model55/1 -> temp_bus_out/55  "temp_sense_55"
  csu_stm_simplified_temperature_model54/1 -> temp_bus_out/54  "temp_sense_54"
  csu_stm_simplified_temperature_model53/1 -> temp_bus_out/53  "temp_sense_53"
  csu_stm_simplified_temperature_model52/1 -> temp_bus_out/52  "temp_sense_52"
  csu_stm_simplified_temperature_model51/1 -> temp_bus_out/51  "temp_sense_51"
  csu_stm_simplified_temperature_model50/1 -> temp_bus_out/50  "temp_sense_50"
  csu_stm_simplified_temperature_model49/1 -> temp_bus_out/49  "temp_sense_49"
  csu_stm_simplified_temperature_model48/1 -> temp_bus_out/48  "temp_sense_48"
  csu_stm_simplified_temperature_model47/1 -> temp_bus_out/47  "temp_sense_47"
  csu_stm_simplified_temperature_model46/1 -> temp_bus_out/46  "temp_sense_46"
  csu_stm_simplified_temperature_model45/1 -> temp_bus_out/45  "temp_sense_45"
  csu_stm_simplified_temperature_model44/1 -> temp_bus_out/44  "temp_sense_44"
  csu_stm_simplified_temperature_model43/1 -> temp_bus_out/43  "temp_sense_43"
  csu_stm_simplified_temperature_model42/1 -> temp_bus_out/42  "temp_sense_42"
  csu_stm_simplified_temperature_model41/1 -> temp_bus_out/41  "temp_sense_41"
  csu_stm_simplified_temperature_model40/1 -> temp_bus_out/40  "temp_sense_40"
  csu_stm_simplified_temperature_model39/1 -> temp_bus_out/39  "temp_sense_39"
  csu_stm_simplified_temperature_model38/1 -> temp_bus_out/38  "temp_sense_38"
  csu_stm_simplified_temperature_model37/1 -> temp_bus_out/37  "temp_sense_37"
  csu_stm_simplified_temperature_model36/1 -> temp_bus_out/36  "temp_sense_36"
  csu_stm_simplified_temperature_model35/1 -> temp_bus_out/35  "temp_sense_35"
  csu_stm_simplified_temperature_model34/1 -> temp_bus_out/34  "temp_sense_34"
  csu_stm_simplified_temperature_model33/1 -> temp_bus_out/33  "temp_sense_33"
  csu_stm_simplified_temperature_model32/1 -> temp_bus_out/32  "temp_sense_32"
  csu_stm_simplified_temperature_model31/1 -> temp_bus_out/31  "temp_sense_31"
  csu_stm_simplified_temperature_model30/1 -> temp_bus_out/30  "temp_sense_30"
  csu_stm_simplified_temperature_model29/1 -> temp_bus_out/29  "temp_sense_29"
  csu_stm_simplified_temperature_model28/1 -> temp_bus_out/28  "temp_sense_28"
  csu_stm_simplified_temperature_model27/1 -> temp_bus_out/27  "temp_sense_27"
  csu_stm_simplified_temperature_model26/1 -> temp_bus_out/26  "temp_sense_26"
  csu_stm_simplified_temperature_model25/1 -> temp_bus_out/25  "temp_sense_25"
  csu_stm_simplified_temperature_model24/1 -> temp_bus_out/24  "temp_sense_24"
  csu_stm_simplified_temperature_model23/1 -> temp_bus_out/23  "temp_sense_23"
  csu_stm_simplified_temperature_model22/1 -> temp_bus_out/22  "temp_sense_22"
  csu_stm_simplified_temperature_model21/1 -> temp_bus_out/21  "temp_sense_21"
  csu_stm_simplified_temperature_model20/1 -> temp_bus_out/20  "temp_sense_20"
  csu_stm_simplified_temperature_model19/1 -> temp_bus_out/19  "temp_sense_19"
  csu_stm_simplified_temperature_model18/1 -> temp_bus_out/18  "temp_sense_18"
  csu_stm_simplified_temperature_model17/1 -> temp_bus_out/17  "temp_sense_17"
  csu_stm_simplified_temperature_model16/1 -> temp_bus_out/16  "temp_sense_16"
  csu_stm_simplified_temperature_model15/1 -> temp_bus_out/15  "temp_sense_15"
  csu_stm_simplified_temperature_model14/1 -> temp_bus_out/14  "temp_sense_14"
  csu_stm_simplified_temperature_model13/1 -> temp_bus_out/13  "temp_sense_13"
  csu_stm_simplified_temperature_model12/1 -> temp_bus_out/12  "temp_sense_12"
  csu_stm_simplified_temperature_model11/1 -> temp_bus_out/11  "temp_sense_11"
  csu_stm_simplified_temperature_model10/1 -> temp_bus_out/10  "temp_sense_10"
  csu_stm_simplified_temperature_model9/1 -> temp_bus_out/9  "temp_sense_9"
  csu_stm_simplified_temperature_model8/1 -> temp_bus_out/8  "temp_sense_8"
  csu_stm_simplified_temperature_model7/1 -> temp_bus_out/7  "temp_sense_7"
  csu_stm_simplified_temperature_model6/1 -> temp_bus_out/6  "temp_sense_6"
  csu_stm_simplified_temperature_model5/1 -> temp_bus_out/5  "temp_sense_5"
  csu_stm_simplified_temperature_model4/1 -> temp_bus_out/4  "temp_sense_4"
  csu_stm_simplified_temperature_model3/1 -> temp_bus_out/3  "temp_sense_3"
  csu_stm_simplified_temperature_model2/1 -> temp_bus_out/2  "temp_sense_2"
  csu_stm_simplified_temperature_model1/1 -> temp_bus_out/1  "temp_sense_1"
